simulink model "task4B_e"  (R2024b)
settings: Solver=VariableStepAuto  StartTime=0.0  StopTime=30  RelTol=1e-3
settings Model: Creator=brope  LastModifiedBy=brope

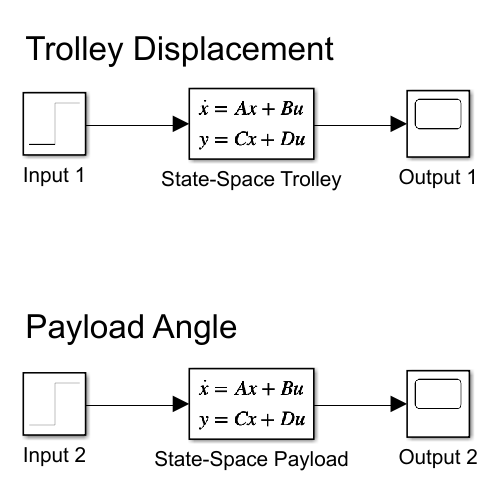
[thumbnail: Simulink's stored preview of the top-level diagram]
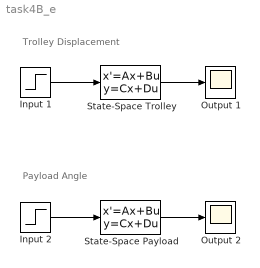
== system task4B_e ==
  note: Trolley Displacement
  note: Payload Angle
  Input 1 : Step  SampleTime=0
  Input 2 : Step  SampleTime=0
  Output 1 : Scope
  Output 2 : Scope
  State-Space Payload : StateSpace  A=[0 1 0 0; 0 0 1 0; 0 0 0 1; 0 -0.02893 -9.4176 -0.007373]  B=[0;0;0;0.005385]  C=[0 0 -1 0]  D=0  InitialCondition=0
  State-Space Trolley : StateSpace  A=[0 1 0 0; 0 0 1 0; 0 0 0 1; 0 -0.02893 -9.4176 -0.007373]  B=[0;0;0;0.005385]  C=[9.81 0 2.5 0]  D=0  InitialCondition=0
  wires:
  Input 2/1 -> State-Space Payload/1
  Input 1/1 -> State-Space Trolley/1
  State-Space Trolley/1 -> Output 1/1
  State-Space Payload/1 -> Output 2/1
